simulink model "velocity_observer"  (R2025a)
settings: Solver=ode15s  StartTime=0.0  StopTime=10.0  FixedStep=0.01  MaxStep=0.01  RelTol=1e-4  AbsTol=1e-7
libraries: robotmaniplib x3, dspsolvers x1
settings Model: Creator=visc1  LastModifiedBy=visc1

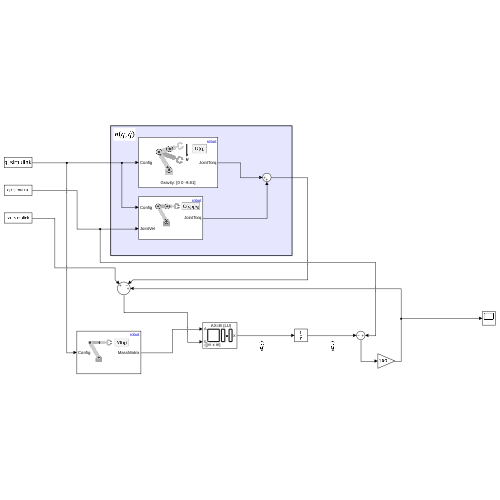
[thumbnail: Simulink's stored preview of the top-level diagram]
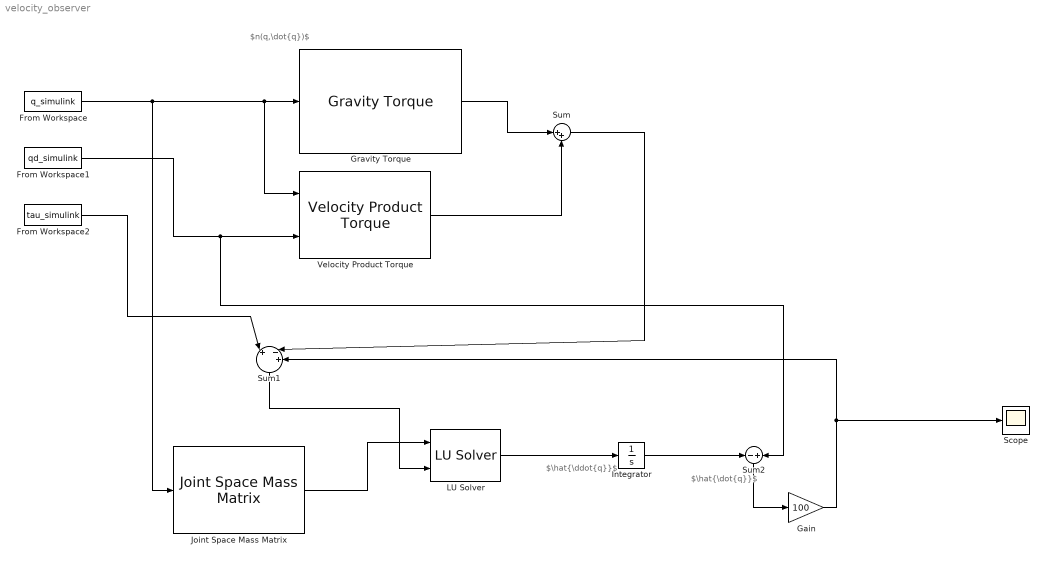
== system velocity_observer ==
  note: $\hat{\ddot{q}}$
  note: $n(q,\dot{q})$
  note: $\hat{\dot{q}}$
  From Workspace : FromWorkspace  VariableName=q_simulink
  From Workspace1 : FromWorkspace  VariableName=qd_simulink
  From Workspace2 : FromWorkspace  VariableName=tau_simulink
  Gain : Gain  Gain=100
  Gravity Torque : robotmaniplib/Gravity Torque  RigidBodyTree=robot  SimulateUsing=Interpreted execution
  Integrator : Integrator
  Joint Space Mass Matrix : robotmaniplib/Joint Space Mass Matrix  RigidBodyTree=robot  SimulateUsing=Interpreted execution
  LU Solver : dspsolvers/LU Solver
  Scope : Scope
      settings: ActiveDisplayYMinimum=-0.094804468860548607  ActiveDisplayYMaximum=0.026357180537147668
  Sum : Sum  Inputs=|++
  Sum1 : Sum  Inputs=|+|-+
  Sum2 : Sum  Inputs=-+
  Velocity Product Torque : robotmaniplib/Velocity Product Torque  RigidBodyTree=robot  SimulateUsing=Interpreted execution
  wires:
  Gravity Torque/1 -> Sum/1
  Velocity Product Torque/1 -> Sum/2
  From Workspace/1 -> Velocity Product Torque/1, Gravity Torque/1, Joint Space Mass Matrix/1
  From Workspace1/1 -> Sum2/2, Velocity Product Torque/2
  From Workspace2/1 -> Sum1/1
  Sum/1 -> Sum1/2
  Joint Space Mass Matrix/1 -> LU Solver/1
  Sum1/1 -> LU Solver/2
  LU Solver/1 -> Integrator/1
  Integrator/1 -> Sum2/1
  Sum2/1 -> Gain/1
  Gain/1 -> Scope/1, Sum1/3
